simulink model "blance_leg"  (R2024b)
settings: Solver=VariableStepAuto  StartTime=0.0  StopTime=13  MaxStep=0.24  RelTol=1e-3
values from neighbouring files (symbols this model uses):
  N = NM + mp*diff(x + L*sin(theta),t,2)    [get_k_length.m]
undefined symbols (not defined in the file or in its folder): a11, a12, a13, a14, a15, a16, a21, a22, a23, a24, a25, a26, X, Y, Z
libraries: sm_lib x102, nesl_utility x22, matrix_library x4, slpidlib x2
(part 1 of 3)
settings Model: SimulationMode=accelerator  Creator=Hhop  LastModifiedBy=21481
settings SolverCC: MinimalZcImpactIntegration=on
settings OptimizationCC: ReuseModelBlockBuffer=off
settings DebuggingCC: ReadBeforeWriteMsg=DisableAll  WriteAfterWriteMsg=DisableAll  WriteAfterReadMsg=DisableAll  MultiTaskDSMMsg=none
settings ModelReferenceCC: UpdateModelReferenceTargets=IfOutOfDate
settings SFSimCC: SFSimEcho=off
settings RTWCC: GPUComputeCapability=3.5

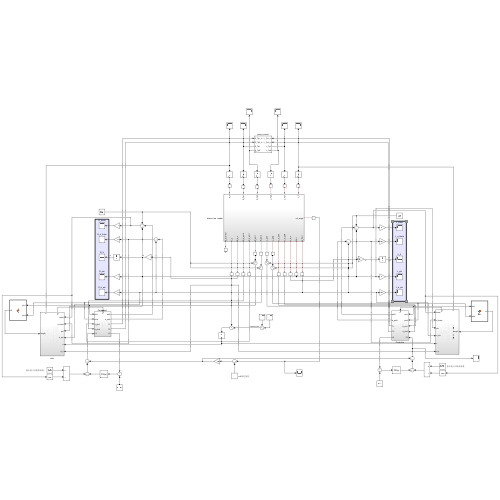
[thumbnail: Simulink's stored preview of the top-level diagram]
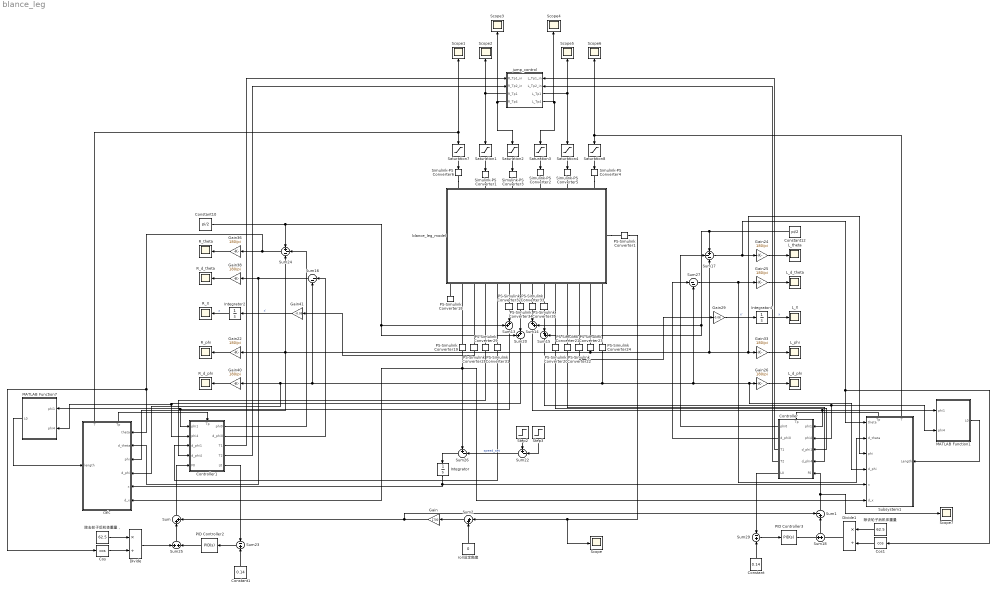
== system blance_leg ==
  Constant : Constant  Value=0.14
  Constant1 : Constant  Value=0.14
  Constant10 : Constant  Value=pi/2
  Constant12 : Constant  Value=pi/2
  Controller : Subsystem
      settings: PortSchema="{\"entries\":[{\"content\":{\"sides\":[{\"content\":{\"connectorIds\":[\"In1\",\"In2\",\"In3\",\"In4\",\"In5\"]},\"type\":\"ConnectorPlacement.EquallySpacedRectSide\",\"uuid\":\"40de31e0-cc19-460f-99e9-affbb47f7204\"},{\"content\":{\"connectorIds\":[\"Out1\",\"Out2\",\"Out3\",\"Out4\",\"Out5\"],\"side\":\"RIGHT\"},\"type\":\"ConnectorPlacement.EquallySpacedRectSide\",\"uuid\":\"e61df4ab-633d-456a-aa2d-223df880274d\"},{\"content\":{\"connectorIds\":[\"In6\"],\"side\":\"TOP\"},\"type\":\"ConnectorPlacement.EquallySpacedRectSide\",\"uuid\":\"a7334146-3144-4ab1-9f08-8bf1583597b4\"}]},\"type\":\"ConnectorPlacement.EquallySpacedConnector\",\"uuid\":\"1490fe93-b025-4c86-96e6-b1bfc13c7f50\"}],\"packageUris\":[\"http://schema.mathworks.com/mf0/Connector/R2020b\"],\"version\":\"1.0\"}"
  Controller1 : Subsystem
      settings: PortSchema="{\"entries\":[{\"content\":{\"sides\":[{\"content\":{\"connectorIds\":[\"In1\",\"In2\",\"In3\",\"In4\",\"In5\"]},\"type\":\"ConnectorPlacement.EquallySpacedRectSide\",\"uuid\":\"40de31e0-cc19-460f-99e9-affbb47f7204\"},{\"content\":{\"connectorIds\":[\"Out1\",\"Out2\",\"Out3\",\"Out4\",\"Out5\"],\"side\":\"RIGHT\"},\"type\":\"ConnectorPlacement.EquallySpacedRectSide\",\"uuid\":\"e61df4ab-633d-456a-aa2d-223df880274d\"},{\"content\":{\"side\":\"TOP\"},\"type\":\"ConnectorPlacement.EquallySpacedRectSide\",\"uuid\":\"a7334146-3144-4ab1-9f08-8bf1583597b4\"},{\"content\":{\"connectorIds\":[\"In6\"],\"side\":\"BOTTOM\"},\"type\":\"ConnectorPlacement.EquallySpacedRectSide\",\"uuid\":\"6688001a-f269-4fa2-b987-774e1f52a18b\"}]},\"type\":\"ConnectorPlacement.EquallySpacedConnector\",\"uuid\":\"1490fe93-b025-4c86-96e6-b1bfc13c7f50\"}],\"packageUris\":[\"http://schema.mathworks.com/mf0/Connector/R2020b\"],\"version\":\"1.0\"}"
  Cos : Trigonometry  Operator=cos
  Cos1 : Trigonometry  Operator=cos
  Divide : Product  Inputs=*/
  Divide1 : Product  Inputs=*/
  Gain : Gain  Gain=1700
  Gain{22,24..26,33,36,38,40} (8 alike) : Gain  Gain=180/pi
  Gain29 : Gain  Gain=-0.06
  Gain41 : Gain  Gain=-0.06
  Integrator : Integrator
  Integrator2 : Integrator
  Integrator4 : Integrator
  L_X : Scope
  L_d_phi : Scope
  L_d_theta : Scope
  L_phi : Scope
  L_theta : Scope
  MATLAB Function1 : MATLAB Function  TreatAsAtomicUnit=on
  MATLAB Function7 : MATLAB Function  TreatAsAtomicUnit=on
  PID Controller2 : slpidlib/PID Controller  Controller=PID  Form=Parallel  TimeDomain=Continuous-time  UseExternalTs=off  SampleTime=-1  IntegratorMethod=Forward Euler  FilterMethod=Forward Euler  ControllerParametersSource=internal  P=500  I=0  UseKiTs=off  D=200  UseExternalDerivativeSource=off  N=100  UseFilter=on  TunerSelectOption=Transfer Function Based (PID Tuner App)  InitialConditionSource=internal  InitialConditionForIntegrator=0  InitialConditionForFilter=0  DifferentiatorICPrevScaledInput=0  ExternalReset=none  TrackingMode=off  Kt=1  LimitOutput=off  SatLimitsSource=internal  UpperSaturationLimit=inf  LowerSaturationLimit=-inf  LinearizeAsGain=on  AntiWindupMode=none  Kb=1  LimitIntegrator=off  UpperIntegratorSaturationLimit=inf  LowerIntegratorSaturationLimit=-inf  POutMin=[]  POutMax=[]  IOutMin=[]  IOutMax=[]  DOutMin=[]  DOutMax=[]  NOutMin=[]  NOutMax=[]  SumOutMin=[]  SumOutMax=[]  SaturationOutMin=[]  SaturationOutMax=[]  PParamMin=[]  PParamMax=[]  IParamMin=[]  IParamMax=[]  DParamMin=[]  DParamMax=[]  NParamMin=[]  NParamMax=[]  KbParamMin=[]  KbParamMax=[]  KtParamMin=[]  KtParamMax=[]  KbOutMin=[]  KbOutMax=[]  KtOutMin=[]  KtOutMax=[]  IntegratorOutMin=[]  IntegratorOutMax=[]  FilterOutMin=[]  FilterOutMax=[]  SumI1OutMin=[]  SumI1OutMax=[]  SumI2OutMin=[]  SumI2OutMax=[]  SumI3OutMin=[]  SumI3OutMax=[]  SumI4OutMin=[]  SumI4OutMax=[]  SumDOutMin=[]  SumDOutMax=[]  DifferentiatorOutMin=[]  DifferentiatorOutMax=[]  FilterDiffOutCoefMin=[]  FilterDiffOutCoefMax=[]  ReciprocalOutMin=[]  ReciprocalOutMax=[]  SumDenOutMin=[]  SumDenOutMax=[]  SumNumOutMin=[]  SumNumOutMax=[]  DivideOutMin=[]  DivideOutMax=[]  UdiffTsProdOutMin=[]  UdiffTsProdOutMax=[]  NTsProdOutMin=[]  NTsProdOutMax=[]  UintegralTsProdOutMin=[]  UintegralTsProdOutMax=[]  UngainTsProdOutMin=[]  UngainTsProdOutMax=[]  ClampingZeroOutDataTypeStr=Inherit: Inherit via back propagation  ClampingZeroOutMin=[]  ClampingZeroOutMax=[]  FilterDenConstantOutDataTypeStr=Inherit: Inherit via back propagation  FilterDenConstantOutMin=[]  FilterDenConstantOutMax=[]  PCopyOutDataTypeStr=Inherit: Inherit via back propagation  PCopyOutMin=[]  PCopyOutMax=[]  NCopyOutDataTypeStr=Inherit: Inherit via back propagation  NCopyOutMin=[]  NCopyOutMax=[]  IntegratorContinuousStateAttributes=''  IntegratorStateMustResolveToSignalObject=off  IntegratorRTWStateStorageClass=Auto  FilterContinuousStateAttributes=''  FilterStateMustResolveToSignalObject=off  FilterRTWStateStorageClass=Auto  ParallelPVariant=InternalParameters  IdealPVariant=Disabled  IVariant=InternalParameters  DVariant=InternalParameters  IntegratorVariant=Continuous  SatVariant=Disabled  AWVariant=Passthrough  PCopyVariant=Disabled  TRVariant=Disabled  FdbkBlocksVariant=Forward  IdealPFdbkVariant=Disabled  SatFdbkVariant=Disabled  DerivativeFilterVariant=ContFilter  NVariant=InternalParameters  NCopyVariant=Disabled  FilterICVariant=InternalICsFilter  IntegratorICVariant=InternalICs  ExternalResetVariant=Disabled  TRSumVariant=Passthrough  SumFdbkVariant=Disabled  SumVariant=Sum_PID  TsampFilterVariant=InternalTs  TsampNgainVariant=Passthrough  TsampIntegralVariant=Disabled_SignalSpec  ExternalSaturationOutDataTypeStr=Inherit: Same as second input  DerivativeSourceVariant=ErrorSignal  PreIntVariant=InternalPreInt
  PID Controller3 : slpidlib/PID Controller  Controller=PID  Form=Parallel  TimeDomain=Continuous-time  UseExternalTs=off  SampleTime=-1  IntegratorMethod=Forward Euler  FilterMethod=Forward Euler  ControllerParametersSource=internal  P=500  I=0  UseKiTs=off  D=200  UseExternalDerivativeSource=off  N=100  UseFilter=on  TunerSelectOption=Transfer Function Based (PID Tuner App)  InitialConditionSource=internal  InitialConditionForIntegrator=0  InitialConditionForFilter=0  DifferentiatorICPrevScaledInput=0  ExternalReset=none  TrackingMode=off  Kt=1  LimitOutput=off  SatLimitsSource=internal  UpperSaturationLimit=inf  LowerSaturationLimit=-inf  LinearizeAsGain=on  AntiWindupMode=none  Kb=1  LimitIntegrator=off  UpperIntegratorSaturationLimit=inf  LowerIntegratorSaturationLimit=-inf  POutMin=[]  POutMax=[]  IOutMin=[]  IOutMax=[]  DOutMin=[]  DOutMax=[]  NOutMin=[]  NOutMax=[]  SumOutMin=[]  SumOutMax=[]  SaturationOutMin=[]  SaturationOutMax=[]  PParamMin=[]  PParamMax=[]  IParamMin=[]  IParamMax=[]  DParamMin=[]  DParamMax=[]  NParamMin=[]  NParamMax=[]  KbParamMin=[]  KbParamMax=[]  KtParamMin=[]  KtParamMax=[]  KbOutMin=[]  KbOutMax=[]  KtOutMin=[]  KtOutMax=[]  IntegratorOutMin=[]  IntegratorOutMax=[]  FilterOutMin=[]  FilterOutMax=[]  SumI1OutMin=[]  SumI1OutMax=[]  SumI2OutMin=[]  SumI2OutMax=[]  SumI3OutMin=[]  SumI3OutMax=[]  SumI4OutMin=[]  SumI4OutMax=[]  SumDOutMin=[]  SumDOutMax=[]  DifferentiatorOutMin=[]  DifferentiatorOutMax=[]  FilterDiffOutCoefMin=[]  FilterDiffOutCoefMax=[]  ReciprocalOutMin=[]  ReciprocalOutMax=[]  SumDenOutMin=[]  SumDenOutMax=[]  SumNumOutMin=[]  SumNumOutMax=[]  DivideOutMin=[]  DivideOutMax=[]  UdiffTsProdOutMin=[]  UdiffTsProdOutMax=[]  NTsProdOutMin=[]  NTsProdOutMax=[]  UintegralTsProdOutMin=[]  UintegralTsProdOutMax=[]  UngainTsProdOutMin=[]  UngainTsProdOutMax=[]  ClampingZeroOutDataTypeStr=Inherit: Inherit via back propagation  ClampingZeroOutMin=[]  ClampingZeroOutMax=[]  FilterDenConstantOutDataTypeStr=Inherit: Inherit via back propagation  FilterDenConstantOutMin=[]  FilterDenConstantOutMax=[]  PCopyOutDataTypeStr=Inherit: Inherit via back propagation  PCopyOutMin=[]  PCopyOutMax=[]  NCopyOutDataTypeStr=Inherit: Inherit via back propagation  NCopyOutMin=[]  NCopyOutMax=[]  IntegratorContinuousStateAttributes=''  IntegratorStateMustResolveToSignalObject=off  IntegratorRTWStateStorageClass=Auto  FilterContinuousStateAttributes=''  FilterStateMustResolveToSignalObject=off  FilterRTWStateStorageClass=Auto  ParallelPVariant=InternalParameters  IdealPVariant=Disabled  IVariant=InternalParameters  DVariant=InternalParameters  IntegratorVariant=Continuous  SatVariant=Disabled  AWVariant=Passthrough  PCopyVariant=Disabled  TRVariant=Disabled  FdbkBlocksVariant=Forward  IdealPFdbkVariant=Disabled  SatFdbkVariant=Disabled  DerivativeFilterVariant=ContFilter  NVariant=InternalParameters  NCopyVariant=Disabled  FilterICVariant=InternalICsFilter  IntegratorICVariant=InternalICs  ExternalResetVariant=Disabled  TRSumVariant=Passthrough  SumFdbkVariant=Disabled  SumVariant=Sum_PID  TsampFilterVariant=InternalTs  TsampNgainVariant=Passthrough  TsampIntegralVariant=Disabled_SignalSpec  ExternalSaturationOutDataTypeStr=Inherit: Same as second input  DerivativeSourceVariant=ErrorSignal  PreIntVariant=InternalPreInt
  PS-Simulink Converter{1,18..24,28..29,31..35} (15 alike) : nesl_utility/PS-Simulink Converter  PhysicalDomain=network_engine_domain  SubClassName=ps_output  LeftPortType=input  RightPortType=output  PseudoPeriodic=off  Frequencies=[]  VectorFormat=inherit  Unit=inherit  AffineConversion=off
  R_X : Scope
  R_d_phi : Scope
  R_d_theta : Scope
  R_phi : Scope
  R_theta : Scope
  Saturation{1..4} (4 alike) : Saturate  UpperLimit=100  LowerLimit=-100
  Saturation7 : Saturate  UpperLimit=9  LowerLimit=-9
  Saturation8 : Saturate  UpperLimit=9  LowerLimit=-9
  Scope{,1..7} (8 alike) : Scope
  Simulink-PS Converter{1..6} (6 alike) : nesl_utility/Simulink-PS Converter  PhysicalDomain=network_engine_domain  SubClassName=ps_input  LeftPortType=input  RightPortType=output  PseudoPeriodic=off  Frequencies=[]  NoiseDistribution=none  NoiseParameters=[]  Unit=1  AffineConversion=off  FilteringAndDerivatives=provide  SimscapeFilterOrder=1  InputFilterTimeConstant=0.001  UdotUserProvided=0
  Step2 : Step  Time=0.8  After=2.5  SampleTime=0
  Step3 : Step  Time=5  After=2.5  SampleTime=0
  Subsystem1 : Subsystem
      settings: PortSchema="{\"entries\":[{\"content\":{\"sides\":[{\"content\":{\"connectorIds\":[\"In1\",\"In2\",\"In3\",\"In4\",\"In5\",\"In6\"]},\"type\":\"ConnectorPlacement.EquallySpacedRectSide\",\"uuid\":\"055cb80c-cd03-4a8d-aef8-6b3df8c72d3f\"},{\"content\":{\"connectorIds\":[\"In7\"],\"side\":\"RIGHT\"},\"type\":\"ConnectorPlacement.EquallySpacedRectSide\",\"uuid\":\"5756fad1-d70f-4a11-a5af-d2f67bfb0d7e\"},{\"content\":{\"connectorIds\":[\"Out1\",\"Out2\"],\"side\":\"TOP\"},\"type\":\"ConnectorPlacement.EquallySpacedRectSide\",\"uuid\":\"9c70cf42-10f8-4525-9406-562484abf580\"}]},\"type\":\"ConnectorPlacement.EquallySpacedConnector\",\"uuid\":\"7084d402-0e44-4d2f-8cc2-1336d196e84d\"}],\"packageUris\":[\"http://schema.mathworks.com/mf0/Connector/R2020b\"],\"version\":\"1.0\"}"
  Sum{,2,14..15} (4 alike) : Sum  Inputs=|++
  Sum1 : Sum  Inputs=-+|
  Sum13 : Sum  Inputs=++|
  Sum16 : Sum  Inputs=|--
  Sum17 : Sum  Inputs=+--
  Sum18 : Sum  Inputs=+|+
  Sum20 : Sum  Inputs=++|
  Sum22 : Sum  Inputs=+-|
  Sum23 : Sum  Inputs=-|+
  Sum24 : Sum  Inputs=+--
  Sum25 : Sum  Inputs=+|+
  Sum26 : Sum  Inputs=+-|
  Sum27 : Sum  Inputs=|--
  Sum29 : Sum  Inputs=-|+
  blance_leg_model : Subsystem
      settings: PortSchema="{\"entries\":[{\"content\":{\"sides\":[{\"content\":{\"connectorIds\":[\"LConn1\",\"LConn2\",\"LConn3\",\"LConn4\",\"LConn5\",\"LConn6\"]},\"type\":\"ConnectorPlacement.EquallySpacedRectSide\",\"uuid\":\"ed635f35-0836-4900-93e3-56fc3520c8de\"},{\"content\":{\"connectorIds\":[\"RConn1\",\"RConn2\",\"RConn3\",\"RConn4\",\"RConn5\",\"RConn6\",\"RConn7\",\"RConn8\",\"RConn9\",\"RConn10\",\"RConn11\",\"RConn12\",\"RConn13\",\"RConn14\"],\"side\":\"RIGHT\"},\"type\":\"ConnectorPlacement.EquallySpacedRectSide\",\"uuid\":\"bb235ec0-defd-4ad9-96f6-8533dab3fbd9\"},{\"content\":{\"connectorIds\":[],\"side\":\"TOP\"},\"type\":\"ConnectorPlacement.EquallySpacedRectSide\",\"uuid\":\"d719db37-8b3a-4344-b330-944fde418334\"},{\"content\":{\"connectorIds\":[\"RConn15\"],\"side\":\"BOTTOM\"},\"type\":\"ConnectorPlacement.EquallySpacedRectSide\",\"uuid\":\"20f9270b-6ab1-4e89-bf00-e838d12c3c13\"}]},\"type\":\"ConnectorPlacement.EquallySpacedConnector\",\"uuid\":\"a2f25b71-0047-4a2d-a238-dad76f034ab1\"}],\"packageUris\":[\"http://schema.mathworks.com/mf0/Connector/R2020b\"],\"version\":\"1.0\"}"
  calc : Subsystem
      settings: PortSchema="{\"entries\":[{\"content\":{\"sides\":[{\"content\":{\"connectorIds\":[\"In1\",\"In2\",\"In3\",\"In4\",\"In5\",\"In6\"]},\"type\":\"ConnectorPlacement.EquallySpacedRectSide\",\"uuid\":\"055cb80c-cd03-4a8d-aef8-6b3df8c72d3f\"},{\"content\":{\"connectorIds\":[\"In7\"],\"side\":\"RIGHT\"},\"type\":\"ConnectorPlacement.EquallySpacedRectSide\",\"uuid\":\"5756fad1-d70f-4a11-a5af-d2f67bfb0d7e\"},{\"content\":{\"connectorIds\":[\"Out1\",\"Out2\"],\"side\":\"TOP\"},\"type\":\"ConnectorPlacement.EquallySpacedRectSide\",\"uuid\":\"9c70cf42-10f8-4525-9406-562484abf580\"}]},\"type\":\"ConnectorPlacement.EquallySpacedConnector\",\"uuid\":\"7084d402-0e44-4d2f-8cc2-1336d196e84d\"}],\"packageUris\":[\"http://schema.mathworks.com/mf0/Connector/R2020b\"],\"version\":\"1.0\"}"
  jump_control : Subsystem  mask{jump_time=5}
      mask prompts: jump_time "跳跃时间"
      settings: PortSchema="{\"entries\":[{\"content\":{\"sides\":[{\"content\":{\"connectorIds\":[\"In1\",\"In2\",\"Out3\",\"Out4\"]},\"type\":\"ConnectorPlacement.EquallySpacedRectSide\",\"uuid\":\"555f1eec-a1f8-4438-898b-242296387de2\"},{\"content\":{\"connectorIds\":[\"In3\",\"In4\",\"Out1\",\"Out2\"],\"side\":\"RIGHT\"},\"type\":\"ConnectorPlacement.EquallySpacedRectSide\",\"uuid\":\"4e34be98-beb2-4e32-b120-d99682746887\"},{\"content\":{\"connectorIds\":[],\"side\":\"TOP\"},\"type\":\"ConnectorPlacement.EquallySpacedRectSide\",\"uuid\":\"2dbe6b4e-143a-4ee5-b634-fdf47ce3ae58\"}]},\"type\":\"ConnectorPlacement.EquallySpacedConnector\",\"uuid\":\"fd4bce8e-8918-4201-9e0d-25b1dfe9d9e9\"}],\"packageUris\":[\"http://schema.mathworks.com/mf0/Connector/R2020b\"],\"version\":\"1.0\"}"
      mask DialogControl ParameterGroupVar Prompt: 参数
  roll设定角度 : Constant  Value=0
  除去轮子后机体重量 : Constant  Value=62.5
  除去轮子后机体重量， : Constant  Value=62.5
  wires:
  Controller/3(T1) -> jump_control/3(L_Tp1_in)
  Constant12/1 -> Sum15/2, Sum14/2, Sum17/1
  Controller/4(T2) -> jump_control/4(L_Tp2_in)
  Sum26/1 -> Integrator/1
  Gain40/1 -> R_d_phi/1
  Constant/1 -> Sum29/2
  PS-Simulink Converter19/1 -> calc/6(d_x), Subsystem1/6(d_x), Sum26/1
  Sum27/1 -> Subsystem1/2(d_theta), Gain25/1
  Step3/1 -> Sum22/2
  Sum14/1 -> MATLAB Function1/1(phi1), Controller/1(phi1)
  Sum23/1 -> PID Controller2/1
  Controller/1(phi0) -> Sum17/2
  Subsystem1/1(Tp) -> Controller/6(Tp)
  calc/1(Tp) -> Controller1/6(Tp)
  PS-Simulink Converter29/1 -> Controller1/2(d_phi4)
  Sum24/1 -> calc/1(theta), Cos/1, Gain36/1
  Saturation1/1 -> Simulink-PS Converter1/1
  Controller1/5(phi0) -> Sum24/2
  Sum17/1 -> Subsystem1/1(theta), Cos1/1, Gain24/1
  Saturation3/1 -> Simulink-PS Converter2/1
  Controller1/1(L0) -> Sum23/1
  PS-Simulink Converter24/1 -> calc/4(d_phi), Gain40/1, Sum16/2, Subsystem1/4(d_phi), Gain26/1, Sum27/2
  Controller1/4(d_phi0) -> Sum16/1
  Gain33/1 -> L_phi/1
  PS-Simulink Converter20/1 -> Controller/3(d_phi1)
  PS-Simulink Converter28/1 -> Gain41/1
  PS-Simulink Converter32/1 -> Sum13/2
  PS-Simulink Converter34/1 -> Sum20/2
  Sum13/1 -> Controller1/5(phi1), MATLAB Function7/1(phi1)
  Sum15/1 -> MATLAB Function1/2(phi4), Controller/2(phi4)
  Controller/5(L0) -> Sum29/1
  PID Controller3/1 -> Sum18/1
  Integrator4/1 -> L_X/1  "x"
  PID Controller2/1 -> Sum25/2
  Gain22/1 -> R_phi/1
  Constant10/1 -> Sum20/1, Sum13/1, Sum24/1
  Integrator2/1 -> R_X/1  "x"
  Sum29/1 -> PID Controller3/1
  Gain26/1 -> L_d_phi/1
  Saturation2/1 -> Simulink-PS Converter3/1
  Sum16/1 -> calc/2(d_theta), Gain38/1
  Gain24/1 -> L_theta/1
  Gain/1 -> Sum1/1, Sum/2
  PS-Simulink Converter1/1 -> Scope/1, Sum2/1
  Sum2/1 -> Gain/1
  roll设定角度/1 -> Sum2/2
  Sum25/1 -> Sum/1
  Subsystem1/2(T) -> Saturation8/1, Scope6/1
  Sum20/1 -> Controller1/4(phi4), MATLAB Function7/2(phi4)
  calc/2(T) -> Saturation7/1, Scope1/1
  Sum18/1 -> Sum1/2
  Gain38/1 -> R_d_theta/1
  jump_control/2(L_Tp4) -> Scope4/1, Saturation3/1
  Step2/1 -> Sum22/1
  Controller1/2(T2) -> jump_control/2(R_Tp2_in)
  Controller/2(d_phi0) -> Sum27/1
  PS-Simulink Converter31/1 -> Controller1/3(d_phi1)
  Gain41/1 -> Integrator2/1  "x'"
  Saturation4/1 -> Simulink-PS Converter5/1
  PS-Simulink Converter33/1 -> Sum14/1
  Controller1/3(T1) -> jump_control/1(R_Tp1_in)
  Sum/1 -> Controller1/1(F0)
  jump_control/1(L_Tp1) -> Saturation4/1, Scope5/1
  PS-Simulink Converter22/1 -> Gain29/1
  PS-Simulink Converter35/1 -> Sum15/1
  PS-Simulink Converter23/1 -> calc/3(phi), Gain22/1, Sum24/3, Subsystem1/3(phi), Gain33/1, Sum17/3
  Saturation7/1 -> Simulink-PS Converter6/1
  Constant1/1 -> Sum23/2
  Saturation8/1 -> Simulink-PS Converter4/1
  Sum1/1 -> Scope7/1, Controller/5(F0)
  Gain36/1 -> R_theta/1
  jump_control/4(R_Tp4) -> Scope3/1, Saturation2/1
  jump_control/3(R_Tp1) -> Saturation1/1, Scope2/1
  Integrator/1 -> Subsystem1/5(x), calc/5(x)
  Gain25/1 -> L_d_theta/1
  Gain29/1 -> Integrator4/1  "x'"
  Sum22/1 -> Sum26/2  "speed_set"
  PS-Simulink Converter21/1 -> Controller/4(d_phi4)
  MATLAB Function1/1(L0) -> Subsystem1/7(Length)
  MATLAB Function7/1(L0) -> calc/7(length)
  除去轮子后机体重量，/1 -> Divide/1
  Cos/1 -> Divide/2
  Divide/1 -> Sum25/1
  Cos1/1 -> Divide1/2
  Divide1/1 -> Sum18/2
  除去轮子后机体重量/1 -> Divide1/1
  connections:
  PS-Simulink Converter31/LConn1 -- blance_leg_model/RConn5
  PS-Simulink Converter21/LConn1 -- blance_leg_model/RConn11
  PS-Simulink Converter18/LConn1 -- blance_leg_model/RConn1
  PS-Simulink Converter34/LConn1 -- blance_leg_model/RConn7
  PS-Simulink Converter33/LConn1 -- blance_leg_model/RConn8
  PS-Simulink Converter32/LConn1 -- blance_leg_model/RConn6
  PS-Simulink Converter19/LConn1 -- blance_leg_model/RConn2
  PS-Simulink Converter20/LConn1 -- blance_leg_model/RConn10
  Simulink-PS Converter3/RConn1 -- blance_leg_model/LConn3
  Simulink-PS Converter1/RConn1 -- blance_leg_model/LConn2
  PS-Simulink Converter29/LConn1 -- blance_leg_model/RConn4
  PS-Simulink Converter22/LConn1 -- blance_leg_model/RConn12
  PS-Simulink Converter28/LConn1 -- blance_leg_model/RConn3
  blance_leg_model/RConn15 -- PS-Simulink Converter1/LConn1
  PS-Simulink Converter35/LConn1 -- blance_leg_model/RConn9
  Simulink-PS Converter2/RConn1 -- blance_leg_model/LConn4
  Simulink-PS Converter5/RConn1 -- blance_leg_model/LConn5
  PS-Simulink Converter24/LConn1 -- blance_leg_model/RConn14
  PS-Simulink Converter23/LConn1 -- blance_leg_model/RConn13
  Simulink-PS Converter6/RConn1 -- blance_leg_model/LConn1
  Simulink-PS Converter4/RConn1 -- blance_leg_model/LConn6

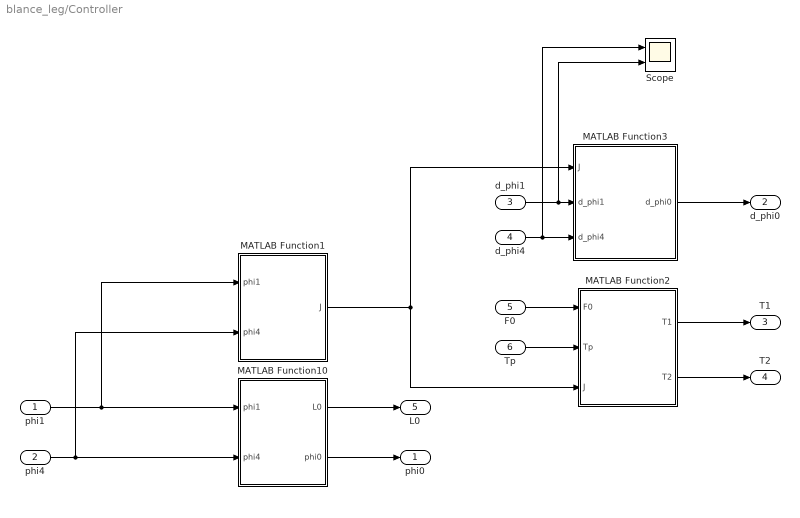
== system blance_leg/Controller ==
  phi1 : Inport
  phi4 : Inport  Port=2
  d_phi1 : Inport  Port=3
  d_phi4 : Inport  Port=4
  F0 : Inport  Port=5
  Tp : Inport  Port=6
  MATLAB Function1 : MATLAB Function  TreatAsAtomicUnit=on
  MATLAB Function10 : MATLAB Function  TreatAsAtomicUnit=on
  MATLAB Function2 : MATLAB Function  TreatAsAtomicUnit=on
  MATLAB Function3 : MATLAB Function  TreatAsAtomicUnit=on
  Scope : Scope  NumInputPorts=2
  phi0 : Outport
  d_phi0 : Outport  Port=2
  T1 : Outport  Port=3
  T2 : Outport  Port=4
  L0 : Outport  Port=5
  wires:
  phi1/1 -> MATLAB Function1/1(phi1), MATLAB Function10/1(phi1)
  MATLAB Function10/2(phi0) -> phi0/1
  phi4/1 -> MATLAB Function1/2(phi4), MATLAB Function10/2(phi4)
  MATLAB Function10/1(L0) -> L0/1
  MATLAB Function1/1(J) -> MATLAB Function2/3(J), MATLAB Function3/1(J)
  MATLAB Function2/1(T1) -> T1/1
  MATLAB Function2/2(T2) -> T2/1
  MATLAB Function3/1(d_phi0) -> d_phi0/1
  Tp/1 -> MATLAB Function2/2(Tp)
  F0/1 -> MATLAB Function2/1(F0)
  d_phi1/1 -> Scope/2, MATLAB Function3/2(d_phi1)
  d_phi4/1 -> Scope/1, MATLAB Function3/3(d_phi4)

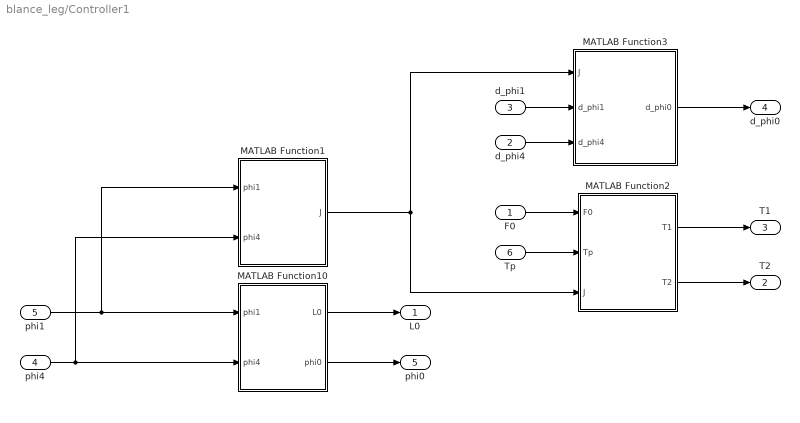
== system blance_leg/Controller1 ==
  F0 : Inport
  d_phi4 : Inport  Port=2
  d_phi1 : Inport  Port=3
  phi4 : Inport  Port=4
  phi1 : Inport  Port=5
  Tp : Inport  Port=6
  MATLAB Function1 : MATLAB Function  TreatAsAtomicUnit=on
  MATLAB Function10 : MATLAB Function  TreatAsAtomicUnit=on
  MATLAB Function2 : MATLAB Function  TreatAsAtomicUnit=on
  MATLAB Function3 : MATLAB Function  TreatAsAtomicUnit=on
  L0 : Outport
  T2 : Outport  Port=2
  T1 : Outport  Port=3
  d_phi0 : Outport  Port=4
  phi0 : Outport  Port=5
  wires:
  phi1/1 -> MATLAB Function1/1(phi1), MATLAB Function10/1(phi1)
  MATLAB Function10/2(phi0) -> phi0/1
  phi4/1 -> MATLAB Function1/2(phi4), MATLAB Function10/2(phi4)
  MATLAB Function10/1(L0) -> L0/1
  MATLAB Function1/1(J) -> MATLAB Function2/3(J), MATLAB Function3/1(J)
  MATLAB Function2/1(T1) -> T1/1
  MATLAB Function2/2(T2) -> T2/1
  MATLAB Function3/1(d_phi0) -> d_phi0/1
  Tp/1 -> MATLAB Function2/2(Tp)
  F0/1 -> MATLAB Function2/1(F0)
  d_phi1/1 -> MATLAB Function3/2(d_phi1)
  d_phi4/1 -> MATLAB Function3/3(d_phi4)

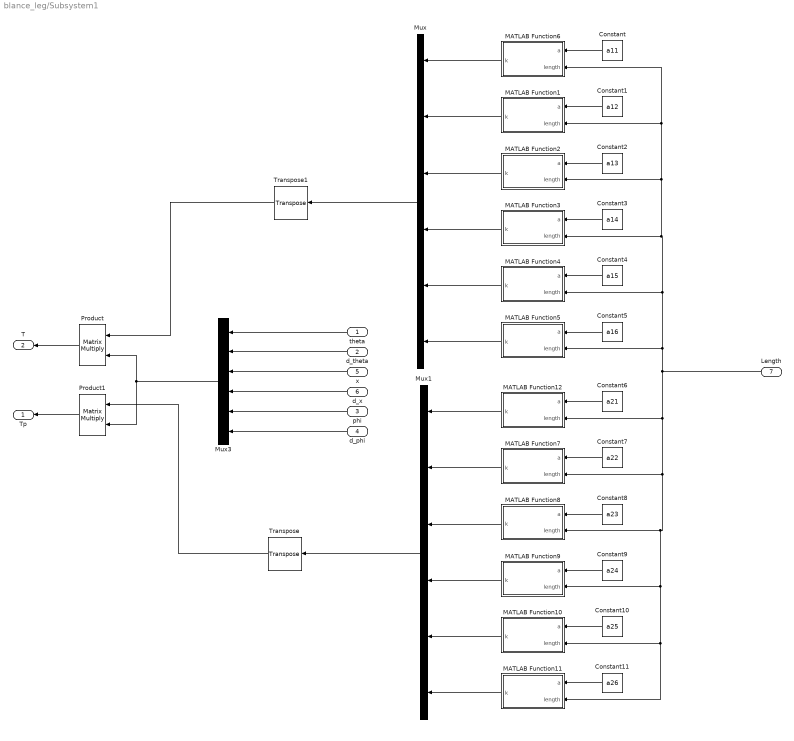
== system blance_leg/Subsystem1 ==
  theta : Inport
  d_theta : Inport  Port=2
  phi : Inport  Port=3
  d_phi : Inport  Port=4
  x : Inport  Port=5
  d_x : Inport  Port=6
  Length : Inport  Port=7
  Constant : Constant  Value=a11
  Constant1 : Constant  Value=a12
  Constant10 : Constant  Value=a25
  Constant11 : Constant  Value=a26
  Constant2 : Constant  Value=a13
  Constant3 : Constant  Value=a14
  Constant4 : Constant  Value=a15
  Constant5 : Constant  Value=a16
  Constant6 : Constant  Value=a21
  Constant7 : Constant  Value=a22
  Constant8 : Constant  Value=a23
  Constant9 : Constant  Value=a24
  MATLAB Function1 : MATLAB Function  TreatAsAtomicUnit=on
  MATLAB Function10 : MATLAB Function  TreatAsAtomicUnit=on
  MATLAB Function11 : MATLAB Function  TreatAsAtomicUnit=on
  MATLAB Function12 : MATLAB Function  TreatAsAtomicUnit=on
  MATLAB Function2 : MATLAB Function  TreatAsAtomicUnit=on
  MATLAB Function3 : MATLAB Function  TreatAsAtomicUnit=on
  MATLAB Function4 : MATLAB Function  TreatAsAtomicUnit=on
  MATLAB Function5 : MATLAB Function  TreatAsAtomicUnit=on
  MATLAB Function6 : MATLAB Function  TreatAsAtomicUnit=on
  MATLAB Function7 : MATLAB Function  TreatAsAtomicUnit=on
  MATLAB Function8 : MATLAB Function  TreatAsAtomicUnit=on
  MATLAB Function9 : MATLAB Function  TreatAsAtomicUnit=on
  Mux : Mux  Inputs=6
  Mux1 : Mux  Inputs=6
  Mux3 : Mux  Inputs=6
  Product : Product  Multiplication=Matrix(*)
  Product1 : Product  Multiplication=Matrix(*)
  Transpose : matrix_library/Transpose
  Transpose1 : matrix_library/Transpose
  Tp : Outport
  T : Outport  Port=2
  wires:
  theta/1 -> Mux3/1
  d_theta/1 -> Mux3/2
  d_x/1 -> Mux3/4
  d_phi/1 -> Mux3/6
  phi/1 -> Mux3/5
  x/1 -> Mux3/3
  Length/1 -> MATLAB Function9/2(length), MATLAB Function10/2(length), MATLAB Function11/2(length), MATLAB Function8/2(length), MATLAB Function7/2(length), MATLAB Function12/2(length), MATLAB Function6/2(length), MATLAB Function1/2(length), MATLAB Function2/2(length), MATLAB Function3/2(length), MATLAB Function4/2(length), MATLAB Function5/2(length)
  MATLAB Function2/1(k) -> Mux/3
  MATLAB Function10/1(k) -> Mux1/5
  MATLAB Function5/1(k) -> Mux/6
  Constant9/1 -> MATLAB Function9/1(a)
  Constant8/1 -> MATLAB Function8/1(a)
  Constant10/1 -> MATLAB Function10/1(a)
  MATLAB Function12/1(k) -> Mux1/1
  MATLAB Function6/1(k) -> Mux/1
  MATLAB Function1/1(k) -> Mux/2
  MATLAB Function11/1(k) -> Mux1/6
  MATLAB Function7/1(k) -> Mux1/2
  Constant6/1 -> MATLAB Function12/1(a)
  Constant1/1 -> MATLAB Function1/1(a)
  Constant7/1 -> MATLAB Function7/1(a)
  Constant5/1 -> MATLAB Function5/1(a)
  Constant3/1 -> MATLAB Function3/1(a)
  Constant11/1 -> MATLAB Function11/1(a)
  Constant2/1 -> MATLAB Function2/1(a)
  MATLAB Function9/1(k) -> Mux1/4
  Constant/1 -> MATLAB Function6/1(a)
  MATLAB Function4/1(k) -> Mux/5
  Constant4/1 -> MATLAB Function4/1(a)
  MATLAB Function3/1(k) -> Mux/4
  MATLAB Function8/1(k) -> Mux1/3
  Mux3/1 -> Product1/2, Product/2
  Mux/1 -> Transpose1/1
  Mux1/1 -> Transpose/1
  Product1/1 -> Tp/1
  Product/1 -> T/1
  Transpose1/1 -> Product/1
  Transpose/1 -> Product1/1
